simulink model "BBB_I2CReadWrite"  (R2013a)
settings: Solver=FixedStepDiscrete  StartTime=0.0  StopTime=inf  FixedStep=0.1  RelTol=1e-3
settings Model: SimulationMode=external  ExtModeTrigDuration=100  Creator=rdustinkahawita  LastModifiedBy=rdustinkahawita
settings OptimizationCC: OptimizeModelRefInitCode=on  LifeSpan=1
settings DebuggingCC: SolverPrmCheckMsg=none  StrictBusMsg=Warning
settings HardwareCC: ProdLargestAtomicInteger=Long  ProdLargestAtomicFloat=Double  ProdEndianess=LittleEndian  ProdHWDeviceType=ARM Compatible->ARM Cortex
settings RTWCC: SystemTargetFile=realtime.tlc  GenerateMakefile=off  TemplateMakefile=realtime.tmf  Description=Run on Target Hardware  RTWVerbose=off  ProcessScript=realtime_make_rtw_hook
settings STFCustomTargetCC: TargetLibSuffix=.a  GenerateSampleERTMain=on  ERTCustomFileBanners=on  SupportNonInlinedSFcns=off  SupportVariableSizeSignals=on  MATLABClassNameForMDSCustomization=Simulink.SoftwareTarget.ERTCustomization  SystemTargetFile=realtime.tlc
settings ERTTargetCC: ParMdlRefBuildCompliant=off  CompOptLevelCompliant=off  ConcurrentExecutionCompliant=off  CombineOutputUpdateFcns=off  ERTFirstTimeCompliant=off  SupportContinuousTime=on  SupportVariableSizeSignals=on  ModelStepFunctionPrototypeControlCompliant=off  CPPClassGenCompliant=off  ExtMode=on  ExtModeMexArgs='192.168.7.2' 0 17725  ERTSrcFileBannerTemplate=realtime_code_template.cgt  ERTHdrFileBannerTemplate=realtime_code_template.cgt  ERTDataSrcFileTemplate=realtime_code_template.cgt  ERTDataHdrFileTemplate=realtime_code_template.cgt  ERTCustomFileTemplate=realtime_file_process.tlc

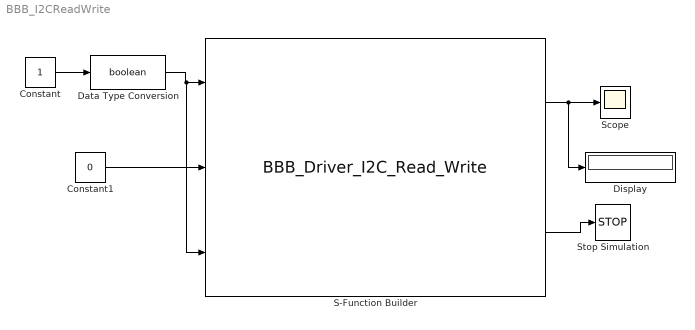
== system BBB_I2CReadWrite ==
  Constant : Constant
  Constant1 : Constant  Value=0  OutDataTypeStr=uint8
  Data Type Conversion : DataTypeConversion  OutMin=[0]  OutMax=[1]  OutDataTypeStr=boolean
  Display : Display
      settings: Format=hex (Stored Integer)
  S-Function Builder : S-Function  InitFcn=try, set_param(gcb,'FunctionName','BBB_Driver_I2C_Read_Write'), end  FunctionName=BBB_Driver_I2C_Read_Write  Parameters=uint8(2),uint8(1),uint8(104),uint8(32),uint8(6)  SFunctionModules=BBB_Driver_I2C_Read_Write_wrapper  EnableBusSupport=off  mask(S-Function Builder){}
      mask help: Simulink:masks:SFunctionBuilder_MD
      mask init:
      | val = [[.9  0.75 0.75 1 1 .9 .9 1]',[1 1 0.75 0.75 .9 .9 1 .9]'];try , sys = get_param(gcb,'SfunBuilderFcnName');if isempty(sys), sys = get_param(gcb,'FunctionName'); end,catch, sys = get_param(gcb,'FunctionName'); end
      settings: CopyFcn=set_param(gcbh,'LinkStatus','none')  PreSaveFcn=try, set_param(gcb,'FunctionName','BBB_Driver_I2C_Read_Write'), end  OpenFcn=sfunctionwizard(gcbh)
      mask Display: plot(val(:,1),val(:,2)),disp(sys), port_label('input',1,'inI2C_WR_Enable'), port_label('input',2,'inI2C_W_Value'), port_label('input',3,'inI2C_WR_Trigger'), port_label('output',1,'outI2C_WR_Data'), port_label('output',2,'outSimStop')
  Scope : Scope
      settings: YMin=102  YMax=102
  Stop Simulation : Stop
  wires:
  Constant/1 -> Data Type Conversion/1
  Data Type Conversion/1 -> S-Function Builder/3, S-Function Builder/1
  Constant1/1 -> S-Function Builder/2
  S-Function Builder/2 -> Stop Simulation/1
  S-Function Builder/1 -> Display/1, Scope/1
